simulink model "computed_torqe_control"  (R2019a)
settings: Solver=ode4  StartTime=0.0  StopTime=2  FixedStep=0.01  RelTol=1e-3
undefined symbols (not defined in the file or in its folder): KI, KP, KV
libraries: simulink x4
settings Model: Creator=JanAriel  LastModifiedBy=JanAriel

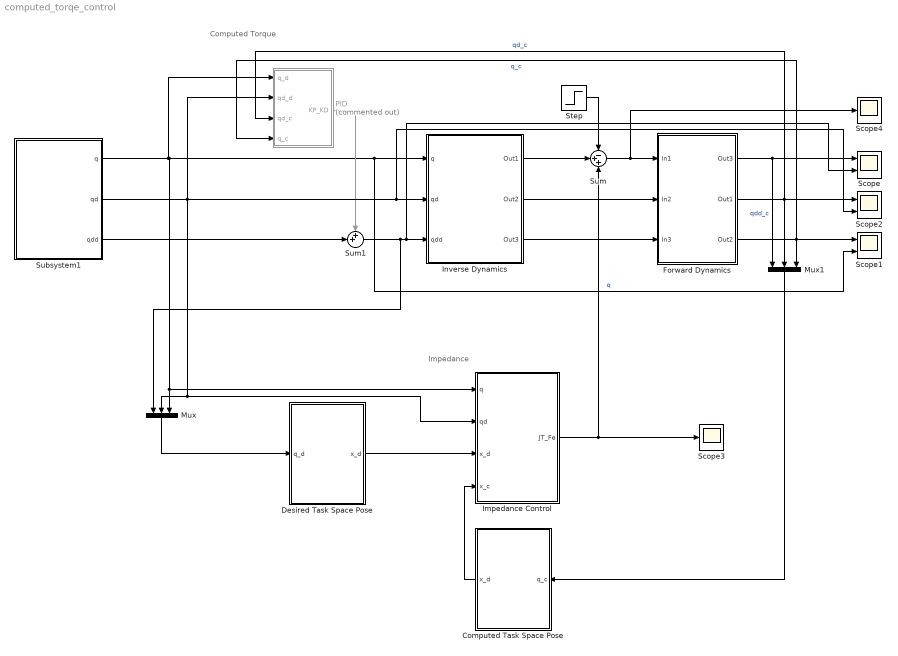
== system computed_torqe_control ==
  note: Impedance
  note: Computed Torque
  Computed Task Space Pose : Subsystem
  Desired Task Space Pose : Subsystem
  Forward Dynamics : Subsystem
  Impedance Control : Subsystem
  Inverse Dynamics : Subsystem
  Mux : Mux  Inputs=3
  Mux1 : Mux  Inputs=3
  PID : Subsystem  Commented=on
  Scope : Scope  NumInputPorts=2
  Scope1 : Scope  NumInputPorts=2
  Scope2 : Scope  NumInputPorts=2
  Scope3 : Scope
  Scope4 : Scope
  Step : Step  Time=0.75  Before=[0;0]  After=[0.2;0.2]  SampleTime=0
  Subsystem1 : Subsystem
  Sum : Sum  Inputs=-++
  Sum1 : Sum  Inputs=++|
  wires:
  Forward Dynamics/2(Out1) -> Scope2/1, PID/3(qd_c), Mux1/2  "qd_c"
  Sum1/1 -> Scope/2, Inverse Dynamics/3(qdd), Mux/1
  Subsystem1/1(q) -> Impedance Control/1(q), Mux/3, Scope1/2, Inverse Dynamics/1(q), PID/1(q_d)  "q"
  Subsystem1/3(qdd) -> Sum1/2
  Inverse Dynamics/2(Out2) -> Forward Dynamics/2(In2)
  Inverse Dynamics/3(Out3) -> Forward Dynamics/3(In3)
  PID/1(KP_KD) -> Sum1/1
  Forward Dynamics/3(Out2) -> Scope1/1, PID/4(q_c), Mux1/3  "q_c"
  Forward Dynamics/1(Out3) -> Scope/1, Mux1/1  "qdd_c"
  Mux/1 -> Desired Task Space Pose/1(q_d)
  Desired Task Space Pose/1(x_d) -> Impedance Control/3(x_d)
  Subsystem1/2(qd) -> Mux/2, Impedance Control/2(qd), Scope2/2, Inverse Dynamics/2(qd), PID/2(qd_d)
  Sum/1 -> Scope4/1, Forward Dynamics/1(In1)
  Inverse Dynamics/1(Out1) -> Sum/2
  Step/1 -> Sum/1
  Mux1/1 -> Computed Task Space Pose/1(q_c)
  Impedance Control/1(JT_Fe) -> Sum/3, Scope3/1
  Computed Task Space Pose/1(x_d) -> Impedance Control/4(x_c)

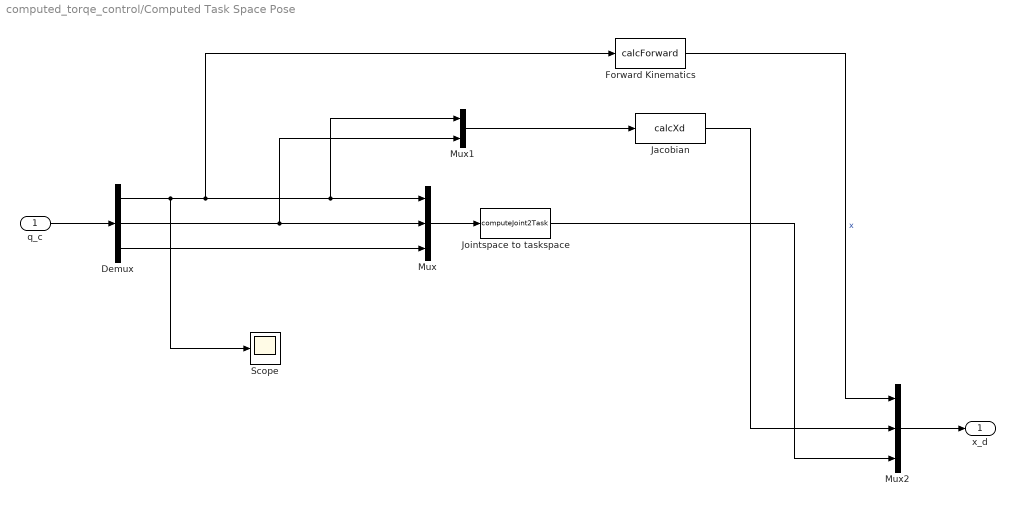
== system computed_torqe_control/Computed Task Space Pose ==
  q_c : Inport
  Demux : Demux  Outputs=3
  Forward Kinematics : MATLABFcn  MATLABFcn=calcForward  Output1D=off
  Jacobian : MATLABFcn  MATLABFcn=calcXd  Output1D=off
  Jointspace to taskspace : MATLABFcn  MATLABFcn=computeJoint2Task  Output1D=off
  Mux : Mux  Inputs=3
  Mux1 : Mux  Inputs=2
  Mux2 : Mux  Inputs=3
  Scope : Scope
  x_d : Outport
  wires:
  q_c/1 -> Demux/1
  Mux/1 -> Jointspace to taskspace/1
  Demux/2 -> Mux1/2, Mux/2
  Forward Kinematics/1 -> Mux2/1  "x"
  Demux/1 -> Scope/1, Forward Kinematics/1, Mux1/1, Mux/1
  Mux1/1 -> Jacobian/1
  Demux/3 -> Mux/3
  Jointspace to taskspace/1 -> Mux2/3
  Jacobian/1 -> Mux2/2
  Mux2/1 -> x_d/1

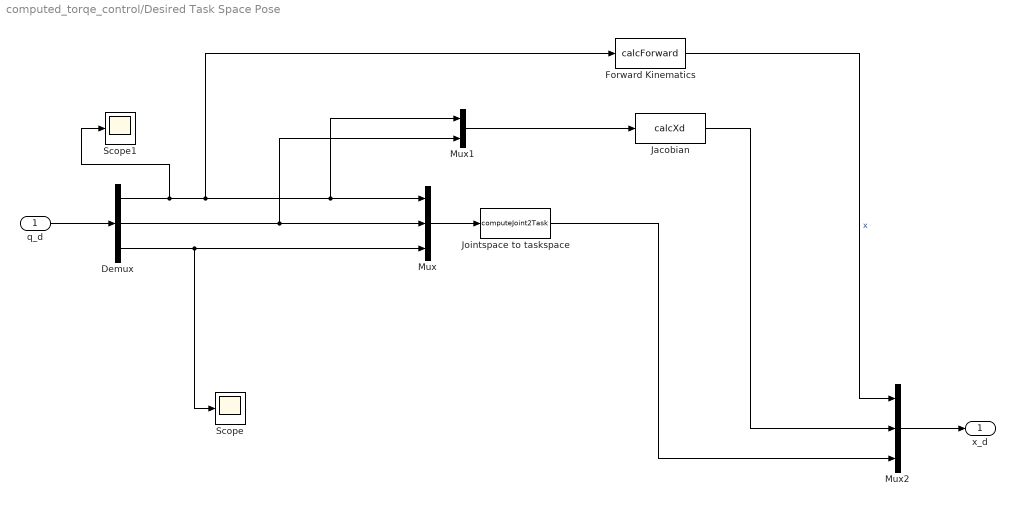
== system computed_torqe_control/Desired Task Space Pose ==
  q_d : Inport
  Demux : Demux  Outputs=3
  Forward Kinematics : MATLABFcn  MATLABFcn=calcForward  Output1D=off
  Jacobian : MATLABFcn  MATLABFcn=calcXd  Output1D=off
  Jointspace to taskspace : MATLABFcn  MATLABFcn=computeJoint2Task  Output1D=off
  Mux : Mux  Inputs=3
  Mux1 : Mux  Inputs=2
  Mux2 : Mux  Inputs=3
  Scope : Scope
  Scope1 : Scope
  x_d : Outport
  wires:
  q_d/1 -> Demux/1
  Mux/1 -> Jointspace to taskspace/1
  Demux/2 -> Mux1/2, Mux/2
  Forward Kinematics/1 -> Mux2/1  "x"
  Mux1/1 -> Jacobian/1
  Demux/3 -> Scope/1, Mux/3
  Jointspace to taskspace/1 -> Mux2/3
  Jacobian/1 -> Mux2/2
  Mux2/1 -> x_d/1
  Demux/1 -> Scope1/1, Forward Kinematics/1, Mux1/1, Mux/1

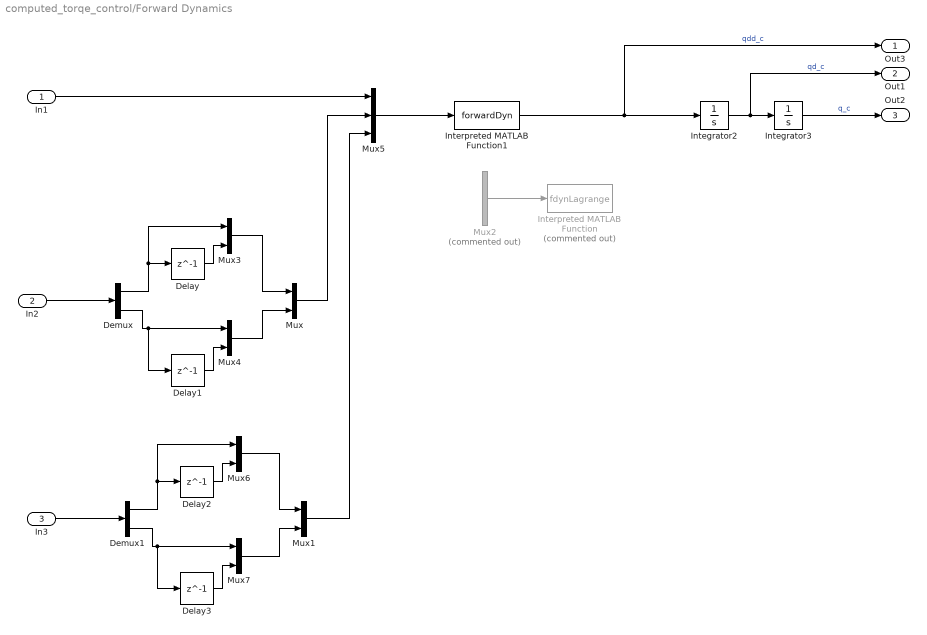
== system computed_torqe_control/Forward Dynamics ==
  In1 : Inport
  In2 : Inport  Port=2
  In3 : Inport  Port=3
  Delay{,1..3} (4 alike) : Delay  DelayLength=1
  Demux : Demux  Outputs=2
  Demux1 : Demux  Outputs=2
  Integrator2 : Integrator
  Integrator3 : Integrator
  Interpreted MATLAB Function : MATLABFcn  Commented=on  MATLABFcn=fdynLagrange  Output1D=off
  Interpreted MATLAB Function1 : MATLABFcn  MATLABFcn=forwardDyn  Output1D=off
  Mux{,1,3..4,6..7} (6 alike) : Mux  Inputs=2
  Mux2 : Mux  Commented=on  Inputs=3
  Mux5 : Mux  Inputs=3
  Out3 : Outport
  Out1 : Outport  Port=2
  Out2 : Outport  Port=3
  wires:
  Integrator2/1 -> Out1/1, Integrator3/1  "qd_c"
  Integrator3/1 -> Out2/1  "q_c"
  Mux5/1 -> Interpreted MATLAB Function1/1
  In2/1 -> Demux/1
  In3/1 -> Demux1/1
  Mux/1 -> Mux5/2
  Mux1/1 -> Mux5/3
  Mux2/1 -> Interpreted MATLAB Function/1
  Interpreted MATLAB Function1/1 -> Out3/1, Integrator2/1  "qdd_c"
  Demux/1 -> Delay/1, Mux3/1
  Delay/1 -> Mux3/2
  Mux3/1 -> Mux/1
  Demux/2 -> Delay1/1, Mux4/1
  Mux4/1 -> Mux/2
  Delay1/1 -> Mux4/2
  Demux1/2 -> Delay3/1, Mux7/1
  Mux6/1 -> Mux1/1
  Delay2/1 -> Mux6/2
  Mux7/1 -> Mux1/2
  Delay3/1 -> Mux7/2
  Demux1/1 -> Delay2/1, Mux6/1
  In1/1 -> Mux5/1

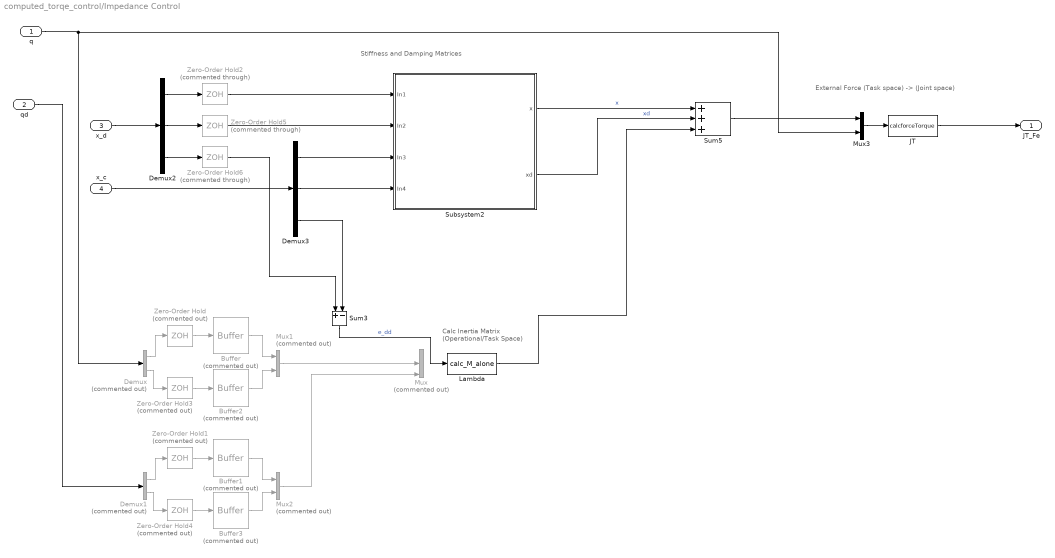
== system computed_torqe_control/Impedance Control ==
  note: External Force (Task space) -> (Joint space)
  note: Stiffness and Damping Matrices
  note: Calc Inertia Matrix (Operational/Task Space)
  q : Inport
  qd : Inport  Port=2
  x_d : Inport  Port=3
  x_c : Inport  Port=4
  Buffer{,1..3} (4 alike) : Buffer  Commented=on  N=2  OutputFrames=off
  Demux : Demux  Commented=on  Outputs=2
  Demux1 : Demux  Commented=on  Outputs=2
  Demux2 : Demux  Outputs=3
  Demux3 : Demux  Outputs=3
  JT : MATLABFcn  MATLABFcn=calcforceTorque  Output1D=off
  Lambda : MATLABFcn  MATLABFcn=calc_M_alone  Output1D=off
  Mux : Mux  Commented=on  Inputs=3
  Mux1 : Mux  Commented=on  Inputs=2
  Mux2 : Mux  Commented=on  Inputs=2
  Mux3 : Mux  Inputs=2
  Subsystem2 : Subsystem
  Sum3 : Sum  Inputs=+-
  Sum5 : Sum  Inputs=+++
  Zero-Order Hold{,1,3..4} (4 alike) : ZeroOrderHold  Commented=on  SampleTime=0.01
  Zero-Order Hold2 : ZeroOrderHold  Commented=through  SampleTime=0.01
  Zero-Order Hold5 : ZeroOrderHold  Commented=through  SampleTime=0.01
  Zero-Order Hold6 : ZeroOrderHold  Commented=through  SampleTime=0.01
  JT_Fe : Outport
  wires:
  Buffer1/1 -> Mux2/1
  Demux1/1 -> Zero-Order Hold1/1
  Sum5/1 -> Mux3/1
  Mux1/1 -> Mux/2
  Sum3/1 -> Lambda/1  "e_dd"
  q/1 -> Demux/1, Mux3/2
  Zero-Order Hold/1 -> Buffer/1
  Buffer/1 -> Mux1/1
  Zero-Order Hold5/1 -> Subsystem2/2(In2)
  Zero-Order Hold4/1 -> Buffer3/1
  Zero-Order Hold1/1 -> Buffer1/1
  Lambda/1 -> Sum5/3
  Buffer3/1 -> Mux2/2
  Buffer2/1 -> Mux1/2
  Zero-Order Hold3/1 -> Buffer2/1
  Demux1/2 -> Zero-Order Hold4/1
  Demux/2 -> Zero-Order Hold3/1
  Zero-Order Hold6/1 -> Sum3/1
  Demux/1 -> Zero-Order Hold/1
  Mux2/1 -> Mux/3
  Mux3/1 -> JT/1
  x_d/1 -> Demux2/1
  JT/1 -> JT_Fe/1
  qd/1 -> Demux1/1
  Zero-Order Hold2/1 -> Subsystem2/1(In1)
  Subsystem2/2(xd) -> Sum5/2  "xd"
  Subsystem2/1(x) -> Sum5/1  "x"
  Demux2/1 -> Zero-Order Hold2/1
  Demux2/2 -> Zero-Order Hold5/1
  Demux2/3 -> Zero-Order Hold6/1
  Demux3/1 -> Subsystem2/3(In3)
  x_c/1 -> Demux3/1
  Demux3/2 -> Subsystem2/4(In4)
  Demux3/3 -> Sum3/2

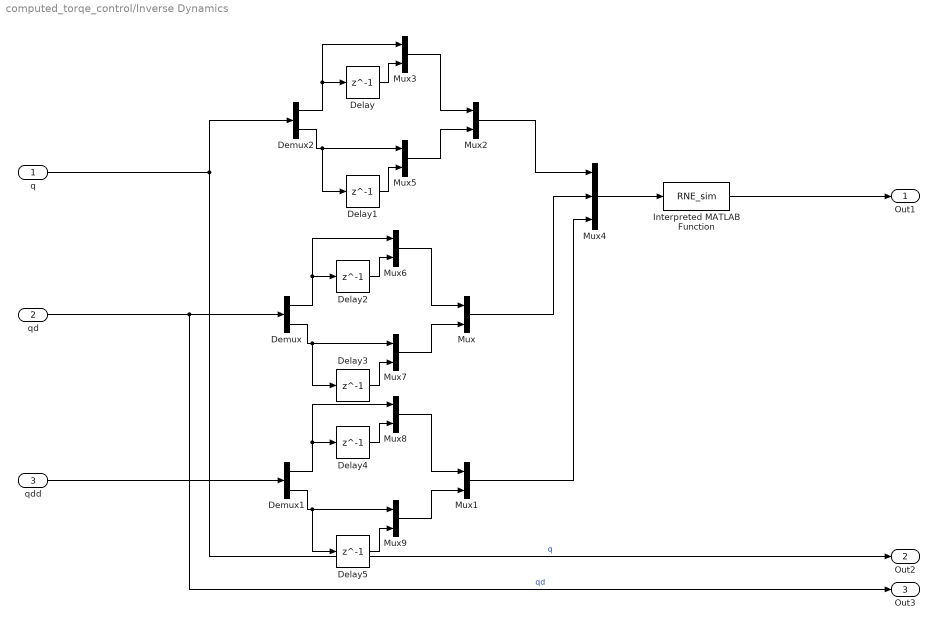
== system computed_torqe_control/Inverse Dynamics ==
  q : Inport
  qd : Inport  Port=2
  qdd : Inport  Port=3
  Delay{,1..5} (6 alike) : Delay  DelayLength=1
  Demux : Demux  Outputs=2
  Demux1 : Demux  Outputs=2
  Demux2 : Demux  Outputs=2
  Interpreted MATLAB Function : MATLABFcn  MATLABFcn=RNE_sim  Output1D=off
  Mux{,1..3,5..9} (9 alike) : Mux  Inputs=2
  Mux4 : Mux  Inputs=3
  Out1 : Outport
  Out2 : Outport  Port=2
  Out3 : Outport  Port=3
  wires:
  qd/1 -> Demux/1, Out3/1  "qd"
  Mux4/1 -> Interpreted MATLAB Function/1
  Interpreted MATLAB Function/1 -> Out1/1
  Mux1/1 -> Mux4/3
  Mux/1 -> Mux4/2
  qdd/1 -> Demux1/1
  Mux2/1 -> Mux4/1
  q/1 -> Out2/1, Demux2/1  "q"
  Demux2/2 -> Delay1/1, Mux5/1
  Mux3/1 -> Mux2/1
  Delay/1 -> Mux3/2
  Mux5/1 -> Mux2/2
  Delay1/1 -> Mux5/2
  Demux2/1 -> Delay/1, Mux3/1
  Demux/2 -> Delay3/1, Mux7/1
  Mux6/1 -> Mux/1
  Delay2/1 -> Mux6/2
  Mux7/1 -> Mux/2
  Delay3/1 -> Mux7/2
  Demux/1 -> Delay2/1, Mux6/1
  Demux1/1 -> Delay4/1, Mux8/1
  Mux9/1 -> Mux1/2
  Demux1/2 -> Delay5/1, Mux9/1
  Delay4/1 -> Mux8/2
  Delay5/1 -> Mux9/2
  Mux8/1 -> Mux1/1

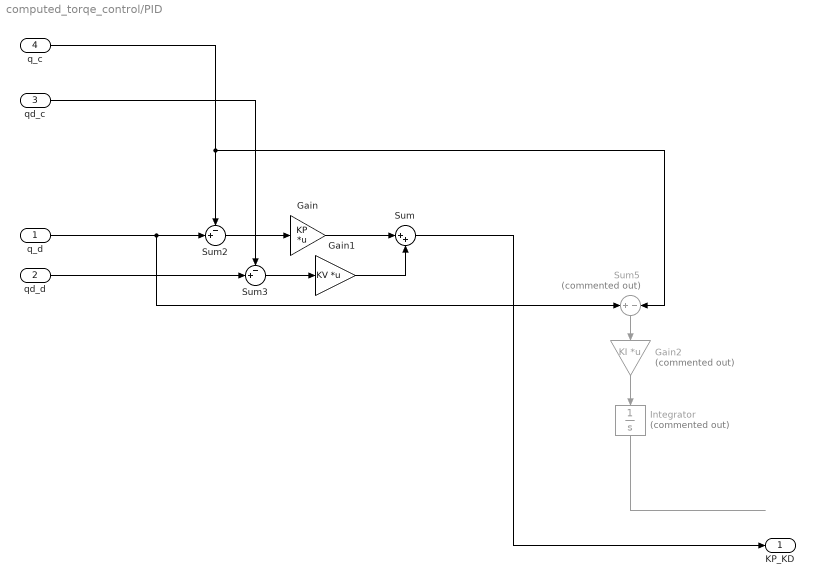
== system computed_torqe_control/PID ==
  q_d : Inport
  qd_d : Inport  Port=2
  qd_c : Inport  Port=3
  q_c : Inport  Port=4
  Gain : Gain  Gain=KP  Multiplication=Matrix(K*u) (u vector)
  Gain1 : Gain  Gain=KV  Multiplication=Matrix(K*u) (u vector)
  Gain2 : Gain  Commented=on  Gain=KI  Multiplication=Matrix(K*u) (u vector)
  Integrator : Integrator  Commented=on
  Sum : Sum  Inputs=|++
  Sum2 : Sum  Inputs=-+|
  Sum3 : Sum  Inputs=-+|
  Sum5 : Sum  Commented=on  Inputs=+-
  KP_KD : Outport
  wires:
  q_c/1 -> Sum5/2, Sum2/1
  Sum5/1 -> Gain2/1
  q_d/1 -> Sum2/2, Sum5/1
  Sum2/1 -> Gain/1
  Sum3/1 -> Gain1/1
  Gain2/1 -> Integrator/1
  Gain1/1 -> Sum/2
  Gain/1 -> Sum/1
  qd_c/1 -> Sum3/1
  Sum/1 -> KP_KD/1
  Integrator/1 -> ?
  qd_d/1 -> Sum3/2

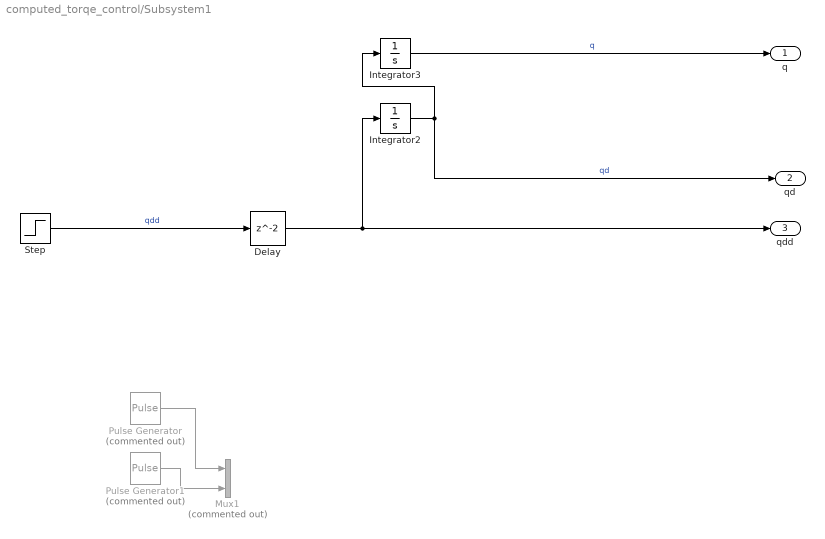
== system computed_torqe_control/Subsystem1 ==
  Delay : Delay
  Integrator2 : Integrator
  Integrator3 : Integrator
  Mux1 : Mux  Commented=on  Inputs=2
  Pulse Generator : DiscretePulseGenerator  Commented=on  PulseType=Time based  PulseWidth=5
  Pulse Generator1 : DiscretePulseGenerator  Commented=on  PulseType=Time based  PulseWidth=5
  Step : Step  Time=0.5  Before=[0;0]  After=[0.35;0.35]  SampleTime=0  VectorParams1D=off
  q : Outport
  qd : Outport  Port=2
  qdd : Outport  Port=3
  wires:
  Integrator2/1 -> qd/1, Integrator3/1  "qd"
  Step/1 -> Delay/1  "qdd"
  Integrator3/1 -> q/1  "q"
  Pulse Generator1/1 -> Mux1/2
  Pulse Generator/1 -> Mux1/1
  Delay/1 -> Integrator2/1, qdd/1

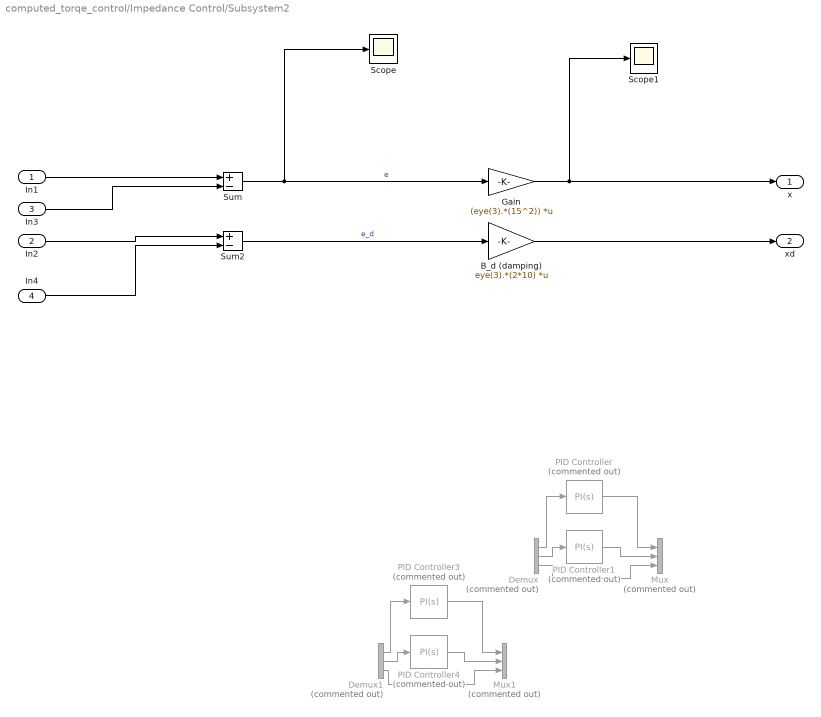
== system computed_torqe_control/Impedance Control/Subsystem2 ==
  In1 : Inport
  In2 : Inport  Port=2
  In3 : Inport  Port=3
  In4 : Inport  Port=4
  B_d (damping) : Gain  Gain=eye(3).*(2*10)  Multiplication=Matrix(K*u) (u vector)
  Demux : Demux  Commented=on  Outputs=3
  Demux1 : Demux  Commented=on  Outputs=3
  Gain : Gain  Gain=(eye(3).*(15^2))  Multiplication=Matrix(K*u) (u vector)
  Mux : Mux  Commented=on  Inputs=3
  Mux1 : Mux  Commented=on  Inputs=3
  PID Controller{,1,3..4} (4 alike) : simulink/Continuous/PID Controller  Commented=on  Controller=PI  Form=Parallel  TimeDomain=Continuous-time  SampleTime=-1  IntegratorMethod=Forward Euler  FilterMethod=Forward Euler  ControllerParametersSource=internal  P=10  I=5  D=0  UseFilter=on  N=100  TunerSelectOption=Transfer Function Based (PID Tuner App)  InitialConditionSource=internal  InitialConditionForIntegrator=0  InitialConditionForFilter=0  DifferentiatorICPrevScaledInput=0  ExternalReset=none  TrackingMode=off  Kt=1  LimitOutput=off  UpperSaturationLimit=inf  LowerSaturationLimit=-inf  LinearizeAsGain=on  AntiWindupMode=none  Kb=1  POutMin=[]  POutMax=[]  IOutMin=[]  IOutMax=[]  DOutMin=[]  DOutMax=[]  NOutMin=[]  NOutMax=[]  SumOutMin=[]  SumOutMax=[]  SaturationOutMin=[]  SaturationOutMax=[]  PParamMin=[]  PParamMax=[]  IParamMin=[]  IParamMax=[]  DParamMin=[]  DParamMax=[]  NParamMin=[]  NParamMax=[]  KbParamMin=[]  KbParamMax=[]  KtParamMin=[]  KtParamMax=[]  KbOutMin=[]  KbOutMax=[]  KtOutMin=[]  KtOutMax=[]  IntegratorOutMin=[]  IntegratorOutMax=[]  FilterOutMin=[]  FilterOutMax=[]  SumI1OutMin=[]  SumI1OutMax=[]  SumI2OutMin=[]  SumI2OutMax=[]  SumI3OutMin=[]  SumI3OutMax=[]  SumI4OutMin=[]  SumI4OutMax=[]  SumDOutMin=[]  SumDOutMax=[]  DifferentiatorOutMin=[]  DifferentiatorOutMax=[]  FilterDiffOutCoefMin=[]  FilterDiffOutCoefMax=[]  ReciprocalOutMin=[]  ReciprocalOutMax=[]  SumDenOutMin=[]  SumDenOutMax=[]  SumNumOutMin=[]  SumNumOutMax=[]  DivideOutMin=[]  DivideOutMax=[]  IntegratorContinuousStateAttributes=''  IntegratorStateMustResolveToSignalObject=off  IntegratorRTWStateStorageClass=Auto  FilterContinuousStateAttributes=''  FilterStateMustResolveToSignalObject=off  FilterRTWStateStorageClass=Auto  ParallelPVariant=InternalParameters  IdealPVariant=Disabled  IVariant=InternalParameters  DVariant=Disabled  IntegratorVariant=Continuous  SatVariant=Disabled  AWVariant=Passthrough  PCopyVariant=Disabled  TRVariant=Disabled  FdbkBlocksVariant=Forward  IdealPFdbkVariant=Disabled  SatFdbkVariant=Disabled  DerivativeFilterVariant=Disabled  NVariant=Disabled  NCopyVariant=Disabled_SignalSpec  FilterICVariant=Disabled  IntegratorICVariant=InternalICs  ExternalResetVariant=Disabled  TRSumVariant=Passthrough  SumFdbkVariant=Disabled  SumVariant=Sum_PI
  Scope : Scope
  Scope1 : Scope
  Sum : Sum  Inputs=+-
  Sum2 : Sum  Inputs=+-
  x : Outport
  xd : Outport  Port=2
  wires:
  Sum/1 -> Gain/1, Scope/1  "e"
  In3/1 -> Sum/2
  In1/1 -> Sum/1
  In4/1 -> Sum2/2
  In2/1 -> Sum2/1
  B_d (damping)/1 -> xd/1
  Gain/1 -> x/1, Scope1/1
  Demux/3 -> Mux/3
  PID Controller1/1 -> Mux/2
  Demux/2 -> PID Controller1/1
  PID Controller/1 -> Mux/1
  Demux/1 -> PID Controller/1
  Demux1/1 -> PID Controller3/1
  PID Controller4/1 -> Mux1/2
  Demux1/2 -> PID Controller4/1
  Demux1/3 -> Mux1/3
  PID Controller3/1 -> Mux1/1
  Sum2/1 -> B_d (damping)/1  "e_d"
